simulink model "CONTROLLER_2"  (R2021a)
settings: Solver=VariableStepAuto  StartTime=0.0  StopTime=inf  RelTol=1e-3
settings Model: DataDictionary=Thermostat.sldd  Creator=smrh1  LastModifiedBy=smrh1

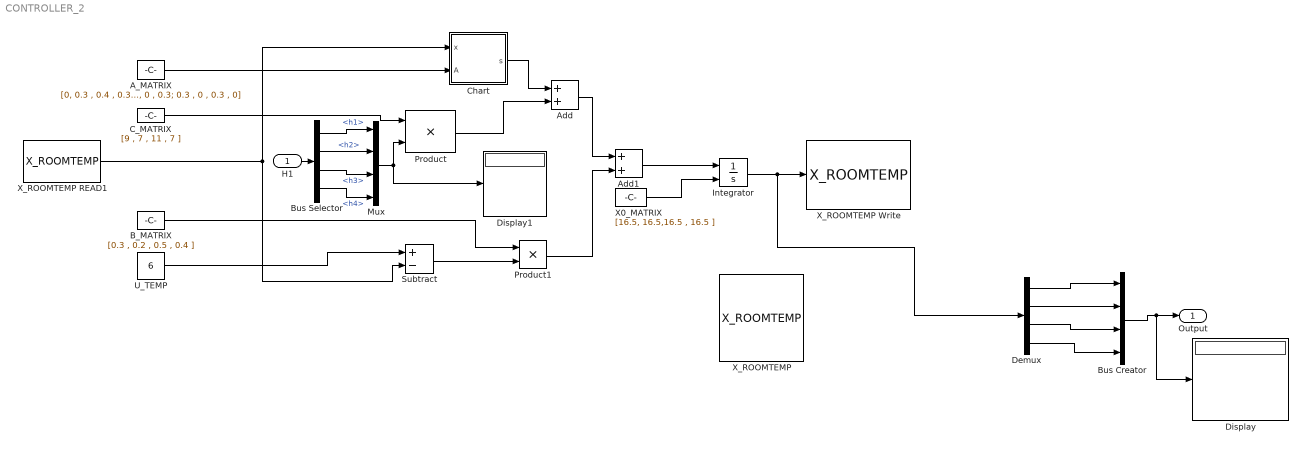
== system CONTROLLER_2 ==
  H1 : Inport  OutDataTypeStr=Bus: Hi
  A_MATRIX : Constant  Value=[0, 0.3 , 0.4 , 0.3 ; 0.3 , 0 , 0.5 , 0 ; 0.4 , 0.5 , 0 , 0.3; 0.3 , 0 , 0.3 , 0]
  Add : Sum
  Add1 : Sum
  B_MATRIX : Constant  Value=[0.3 , 0.2 , 0.5 , 0.4 ]
  Bus Creator : BusCreator  Inputs=4
  Bus Selector : BusSelector  OutputSignals=h1,h2,h3,h4
  C_MATRIX : Constant  Value=[9 , 7 , 11 , 7 ]
  Chart : Stateflow chart  TreatAsAtomicUnit=on
  Demux : Demux
  Display : Display
  Display1 : Display
  Integrator : Integrator  InitialConditionSource=external
  Mux : Mux
  Product : Product
  Product1 : Product
  Subtract : Sum  Inputs=+-
  U_TEMP : Constant  Value=6
  X0_MATRIX : Constant  Value=[16.5, 16.5,16.5 , 16.5 ]
  X_ROOMTEMP : DataStoreMemory  DataStoreName=X_ROOMTEMP  ReadBeforeWriteMsg=warning  WriteAfterWriteMsg=warning  WriteAfterReadMsg=warning  InitialValue=[16.5,16.5,16.5,16.5]  ShowAdditionalParam=off
  X_ROOMTEMP READ1 : DataStoreRead  DataStoreName=X_ROOMTEMP  IndexOptions=Index vector (dialog)  Indices=1  OutputSizes=1
  X_ROOMTEMP Write : DataStoreWrite  DataStoreName=X_ROOMTEMP  IndexOptions=Index vector (dialog)  Indices=1  OutputSizes=1
  Output : Outport  OutDataTypeStr=Bus: Xi
  wires:
  X_ROOMTEMP READ1/1 -> Subtract/2, Chart/1(x)
  U_TEMP/1 -> Subtract/1
  Add/1 -> Add1/1
  X0_MATRIX/1 -> Integrator/2
  A_MATRIX/1 -> Chart/2(A)
  C_MATRIX/1 -> Product/1
  B_MATRIX/1 -> Product1/1
  Subtract/1 -> Product1/2
  Add1/1 -> Integrator/1
  Chart/1(s) -> Add/1
  Product1/1 -> Add1/2
  Product/1 -> Add/2
  H1/1 -> Bus Selector/1
  Demux/1 -> Bus Creator/1
  Demux/2 -> Bus Creator/2
  Demux/3 -> Bus Creator/3
  Demux/4 -> Bus Creator/4
  Bus Creator/1 -> Display/1, Output/1
  Bus Selector/1 -> Mux/1  "<h1>"
  Bus Selector/2 -> Mux/2  "<h2>"
  Bus Selector/3 -> Mux/3  "<h3>"
  Bus Selector/4 -> Mux/4  "<h4>"
  Mux/1 -> Display1/1, Product/2
  Integrator/1 -> Demux/1, X_ROOMTEMP Write/1

== stateflow chart CONTROLLER_2/Chart ==
  state s3
    du:
    s(1) = A(1,2)*(x(2)-x(1)) + A(1,3)*(x(3)-x(1)) + A(1,4)*(x(4)-x(1));
    s(2) = A(2,1)*(x(1)-x(2)) + A(2,3)*(x(3)-x(2)) + A(2,4)*(x(4)-x(2));
    s(3) = A(3,1)*(x(1)-x(3)) + A(3,2)*(x(2)-x(3)) + A(3,4)*(x(4)-x(3));
    s(4) = A(4,1)*(x(1)-x(4)) + A(4,2)*(x(2)-x(4)) + A(4,3)*(x(3)-x(4));
  (default) -> s3 : {s=[0,0,0,0];}
  data: x input; A input; s output
